simulink model "Nyquistbedingungen"  (Simulink 8.6)
settings: Solver=FixedStepDiscrete  StartTime=0  StopTime=inf  RelTol=1e-3
undefined symbols (not defined in the file or in its folder): dfilt, gcbh, magnitude, rcfiltgaincompat
libraries: commfilt2 x12, commrandsrc2 x6, commdigbbndam3 x4, dspobslib x3, dspstat3 x2, commdigbbndpm3 x2, commchan3 x1, dspsigops x1, simulink x1
CloseFcn:
  | rtwprivate ssgencode ModelCloseRequest Nyquist_Bedingungen
settings Model: Creator=schwall  LastModifiedBy=wunsch
settings DataIOCC: SaveOutput=off  SignalLogging=off  SaveTime=off
settings DebuggingCC: FcnCallInpInsideContextMsg=UseLocalSettings

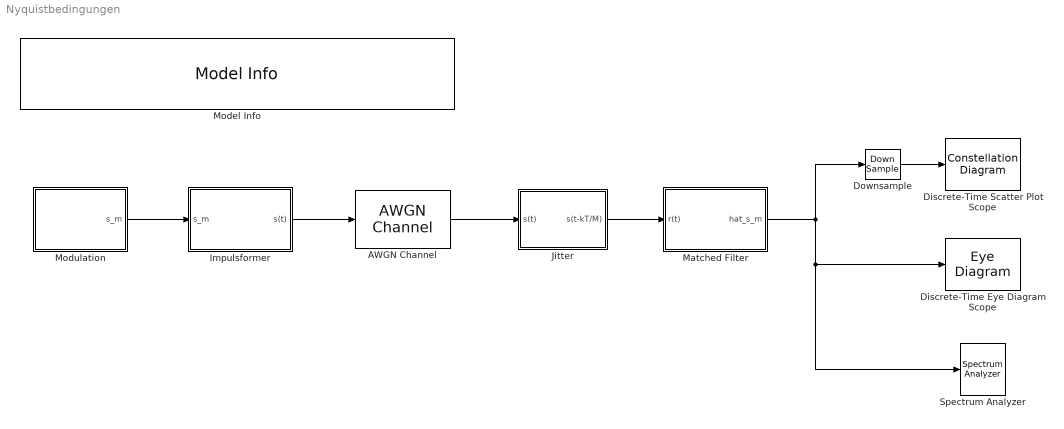
== system Nyquistbedingungen ==
  AWGN Channel : commchan3/AWGN Channel  InputProcessing=Inherited (this choice will be removed - see release notes)  seed=67  noiseMode="Signal to noise ratio  (Es/No)"  EbNodB=10  EsNodB=30  SNRdB=100  bitsPerSym=1  Ps=1/8  Tsym=1/100  variance=1
  Discrete-Time Eye Diagram Scope : EyeDiagram  Tag=EyeDiagram
  Discrete-Time Scatter Plot Scope : ConstellationDiagram  Tag=ScatterPlot
  Downsample : DownSample  N=8
  Impulsformer : Subsystem  mask(Impulsformer){rolloff_set=RRC Rolloff-Faktor 0}
      mask prompts: rolloff_set "Impulsformer:"
      mask help: Impulsformer auswaehlen.
      mask TypeOptions rolloff_set: RRC Rolloff-Faktor 0 | RRC Rolloff-Faktor 0.2 | RRC Rolloff-Faktor 0.4 | RRC Rolloff-Faktor 0.6 | RRC Rolloff-Faktor 0.8 | RRC Rolloff-Faktor 1 | Rechteck-Filter
  Jitter : Subsystem  mask{abtast_set=0}
      mask prompts: abtast_set "Abtastfehler (0...7)"
  Matched Filter : Subsystem  mask(Impulsformer){rolloff_set=RRC Rolloff-Faktor 0}
      mask prompts: rolloff_set "Impulsformer:"
      mask help: Impulsformer auswaehlen.
      mask TypeOptions rolloff_set: RRC Rolloff-Faktor 0 | RRC Rolloff-Faktor 0.2 | RRC Rolloff-Faktor 0.4 | RRC Rolloff-Faktor 0.6 | RRC Rolloff-Faktor 0.8 | RRC Rolloff-Faktor 1 | Rechteck-Filter
  Model Info : simulink/Model-Wide Utilities/Model Info  BlockCM=None  Frame=on  DisplayStringWithTags=|  HorizontalTextAlignment=Left  LeftAlignmentValue=0.02  SourceBlockDiagram=Nyquistbedingungen  TagMaxNumber=20
      | Demo Nyquist Bedingungen
      | Vorlesung Nachrichtentechnik II
      | Institut fuer Nachrichtentechnik (CEL)
  Modulation : Subsystem  mask(Modulation){mod_set=4-QAM, fs=1/100}
      mask prompts: mod_set "Modulationsverfahren:"; fs "Symboldauer [s]"
      mask help: Modulationsverfahren auswaehlen.
      mask TypeOptions mod_set: 2-ASK | QPSK | 16-PSK | 4-QAM | 16-QAM | 256-QAM
  Spectrum Analyzer : SpectrumAnalyzer
  wires:
  Modulation/1(s_m) -> Impulsformer/1(s_m)
  Impulsformer/1(s(t)) -> AWGN Channel/1
  AWGN Channel/1 -> Jitter/1(s(t))
  Downsample/1 -> Discrete-Time Scatter Plot Scope/1
  Matched Filter/1(hat_s_m) -> Downsample/1, Spectrum Analyzer/1, Discrete-Time Eye Diagram Scope/1
  Jitter/1(s(t-kT/M)) -> Matched Filter/1(r(t))

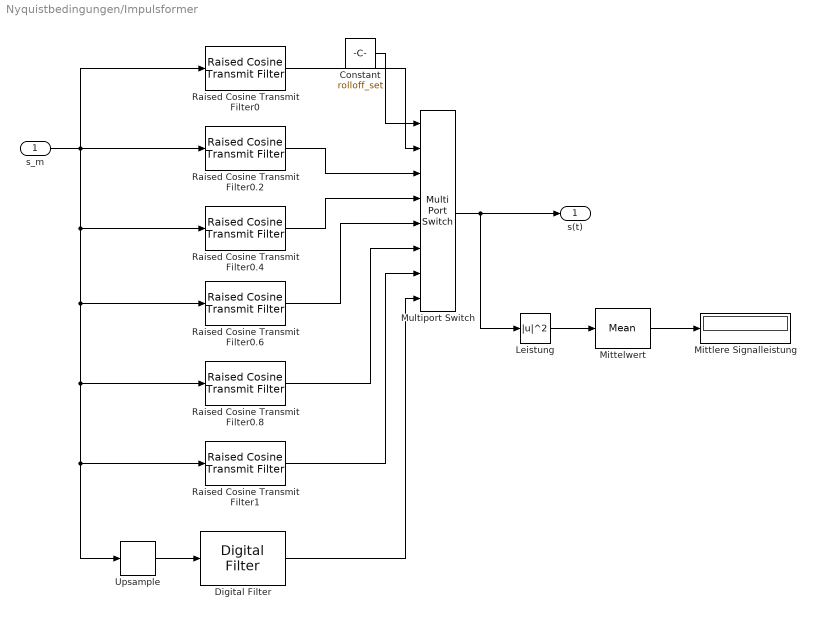
== system Nyquistbedingungen/Impulsformer ==
  s_m : Inport
  Constant : Constant  Value=rolloff_set
  Digital Filter : dspobslib/Digital Filter  TypePopup=FIR (all zeros)  IIRFiltStruct=Direct form II transposed  AllPoleFiltStruct=Direct form  FIRFiltStruct=Direct form  CoeffSource=Specify via dialog  NumCoeffs=1/sqrt(8)*ones(8,1)  DenCoeffs=[1 0.1]  BiQuadCoeffs=[1 0.3 0.4 1 0.1 0.2]  LatticeCoeffs=[0.2 0.4]  denIgnore=on  FiltPerSampPopup=One filter per frame  IC=0  ICnum=0  ICden=0  roundingMode=Floor  overflowMode=off  ScaleValues=1  scaleValueFracLength=14  stageInFracLength=15  stageOutFracLength=15  FilterSource=Specify via dialog  dfiltObjectName=dfilt.dffir([1 2 1])  InputProcessing=Inherited (this choice will be removed - see release notes)
  Leistung : Math  Operator=magnitude^2  SaturateOnIntegerOverflow=on
  Mittelwert : dspstat3/Mean  run=on  reset_popup=None  InputProcessing=Inherited (this choice will be removed - see release notes)  directionMode=Each column  dimension=1  roiEnable=off  roiType=Rectangles  roiPortion=Entire ROI  roiOutput=Individual statistics for each ROI  roiFlag=off  outputDataTypeStr=Inherit: Same as accumulator  outputLastDataTypeStr=Inherit: Same as accumulator  outputMin=[]  outputMax=[]  roundingMode=Floor  overflowMode=off
  Mittlere Signalleistung : Display
  Multiport Switch : MultiPortSwitch  Inputs=7
  Raised Cosine Transmit Filter0 : commfilt2/Raised Cosine Transmit Filter  filtType=Square root  filtSpan=2*(4)  currentFiltSpan=2*(4)  D=4  R=0  sampMode=Mute  saveAsFlag=0  N=8  framing=Maintain input frame rate  InputProcessing=Columns as channels (frame based)  checkGain=User-specified  filterGain=(1)*rcfiltgaincompat(gcbh)  checkCoeff=off  variableName=rcTxFilt  launchFVT=off  roundingMode=Floor  overflowMode=off
  Raised Cosine Transmit Filter0.2 : commfilt2/Raised Cosine Transmit Filter  filtType=Square root  filtSpan=2*(4)  currentFiltSpan=2*(4)  D=4  R=0.2  sampMode=Mute  saveAsFlag=0  N=8  framing=Maintain input frame rate  InputProcessing=Columns as channels (frame based)  checkGain=User-specified  filterGain=(1)*rcfiltgaincompat(gcbh)  checkCoeff=off  variableName=rcTxFilt1  launchFVT=off  roundingMode=Floor  overflowMode=off
  Raised Cosine Transmit Filter0.4 : commfilt2/Raised Cosine Transmit Filter  filtType=Square root  filtSpan=2*(4)  currentFiltSpan=2*(4)  D=4  R=0.4  sampMode=Mute  saveAsFlag=0  N=8  framing=Maintain input frame rate  InputProcessing=Columns as channels (frame based)  checkGain=User-specified  filterGain=(1)*rcfiltgaincompat(gcbh)  checkCoeff=off  variableName=rcTxFilt2  launchFVT=off  roundingMode=Floor  overflowMode=off
  Raised Cosine Transmit Filter0.6 : commfilt2/Raised Cosine Transmit Filter  filtType=Square root  filtSpan=2*(4)  currentFiltSpan=2*(4)  D=4  R=0.6  sampMode=Mute  saveAsFlag=0  N=8  framing=Maintain input frame rate  InputProcessing=Columns as channels (frame based)  checkGain=User-specified  filterGain=(1)*rcfiltgaincompat(gcbh)  checkCoeff=off  variableName=rcTxFilt3  launchFVT=off  roundingMode=Floor  overflowMode=off
  Raised Cosine Transmit Filter0.8 : commfilt2/Raised Cosine Transmit Filter  filtType=Square root  filtSpan=2*(4)  currentFiltSpan=2*(4)  D=4  R=0.8  sampMode=Mute  saveAsFlag=0  N=8  framing=Maintain input frame rate  InputProcessing=Columns as channels (frame based)  checkGain=User-specified  filterGain=(1)*rcfiltgaincompat(gcbh)  checkCoeff=off  variableName=rcTxFilt4  launchFVT=off  roundingMode=Floor  overflowMode=off
  Raised Cosine Transmit Filter1 : commfilt2/Raised Cosine Transmit Filter  filtType=Square root  filtSpan=2*(4)  currentFiltSpan=2*(4)  D=4  R=1  sampMode=Mute  saveAsFlag=0  N=8  framing=Maintain input frame rate  InputProcessing=Columns as channels (frame based)  checkGain=User-specified  filterGain=(1)*rcfiltgaincompat(gcbh)  checkCoeff=off  variableName=rcTxFilt5  launchFVT=off  roundingMode=Floor  overflowMode=off
  Upsample : dspsigops/Upsample  N=8  phase=0  InputProcessing=Inherited (this choice will be removed - see release notes)  RateOptions=Enforce single-rate processing  ic=0  mode=Unused parameter value
  s(t) : Outport
  wires:
  s_m/1 -> Raised Cosine Transmit Filter0/1, Raised Cosine Transmit Filter0.2/1, Raised Cosine Transmit Filter0.4/1, Raised Cosine Transmit Filter0.8/1, Raised Cosine Transmit Filter1/1, Upsample/1, Raised Cosine Transmit Filter0.6/1
  Mittelwert/1 -> Mittlere Signalleistung/1
  Leistung/1 -> Mittelwert/1
  Multiport Switch/1 -> Leistung/1, s(t)/1
  Raised Cosine Transmit Filter0/1 -> Multiport Switch/2
  Raised Cosine Transmit Filter0.2/1 -> Multiport Switch/3
  Raised Cosine Transmit Filter0.4/1 -> Multiport Switch/4
  Raised Cosine Transmit Filter0.6/1 -> Multiport Switch/5
  Raised Cosine Transmit Filter0.8/1 -> Multiport Switch/6
  Raised Cosine Transmit Filter1/1 -> Multiport Switch/7
  Constant/1 -> Multiport Switch/1
  Digital Filter/1 -> Multiport Switch/8
  Upsample/1 -> Digital Filter/1

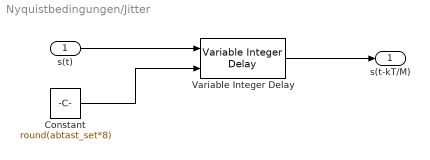
== system Nyquistbedingungen/Jitter ==
  s(t) : Inport
  Constant : Constant  Value=round(abtast_set*8)
  Variable Integer Delay : dspobslib/Variable Integer Delay  dmax=7  InputProcessing=Inherited (this choice will be removed - see release notes)  ic=0  noDFT=off
  s(t-kT/M) : Outport
  wires:
  Variable Integer Delay/1 -> s(t-kT/M)/1
  Constant/1 -> Variable Integer Delay/2
  s(t)/1 -> Variable Integer Delay/1

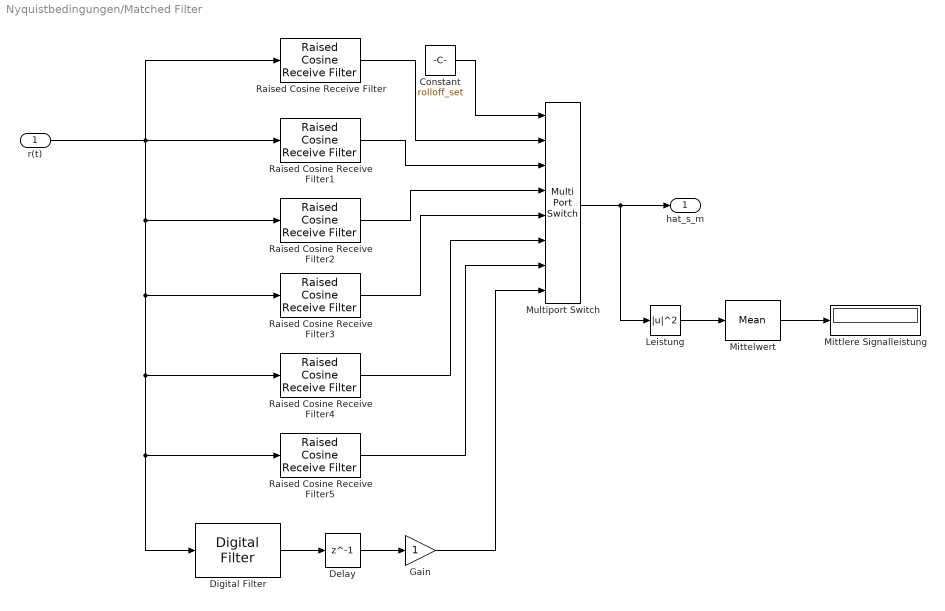
== system Nyquistbedingungen/Matched Filter ==
  r(t) : Inport
  Constant : Constant  Value=rolloff_set
  Delay : Delay  DelayLength=1  InitialCondition=0  InputProcessing=Columns as channels (frame based)
  Digital Filter : dspobslib/Digital Filter  TypePopup=FIR (all zeros)  IIRFiltStruct=Direct form II transposed  AllPoleFiltStruct=Direct form  FIRFiltStruct=Direct form  CoeffSource=Specify via dialog  NumCoeffs=1/sqrt(8)*ones(8,1)  DenCoeffs=[1 0.1]  BiQuadCoeffs=[1 0.3 0.4 1 0.1 0.2]  LatticeCoeffs=[0.2 0.4]  denIgnore=on  FiltPerSampPopup=One filter per frame  IC=0  ICnum=0  ICden=0  roundingMode=Floor  overflowMode=off  ScaleValues=1  scaleValueFracLength=14  stageInFracLength=15  stageOutFracLength=15  FilterSource=Specify via dialog  dfiltObjectName=dfilt.dffir([1 2 1])  InputProcessing=Inherited (this choice will be removed - see release notes)
  Gain : Gain
  Leistung : Math  Operator=magnitude^2  SaturateOnIntegerOverflow=on
  Mittelwert : dspstat3/Mean  run=on  reset_popup=None  InputProcessing=Inherited (this choice will be removed - see release notes)  directionMode=Each column  dimension=1  roiEnable=off  roiType=Rectangles  roiPortion=Entire ROI  roiOutput=Individual statistics for each ROI  roiFlag=off  outputDataTypeStr=Inherit: Same as accumulator  outputLastDataTypeStr=Inherit: Same as accumulator  outputMin=[]  outputMax=[]  roundingMode=Floor  overflowMode=off
  Mittlere Signalleistung : Display
  Multiport Switch : MultiPortSwitch  Inputs=7
  Raised Cosine Receive Filter : commfilt2/Raised Cosine Receive Filter  filtType=Square root  N=8  filtSpan=2*(4)  currentFiltSpan=2*(4)  D=4  R=0  sampMode=Mute  saveAsFlag=0  rateMode=Downsampling  downFactor=1  downOffset=0  framing=Maintain input frame rate  InputProcessing=Columns as channels (frame based)  checkGain=User-specified  filterGain=(1)*rcfiltgaincompat(gcbh)  checkCoeff=off  variableName=rcRxFilt  launchFVT=off  roundingMode=Floor  overflowMode=off
  Raised Cosine Receive Filter1 : commfilt2/Raised Cosine Receive Filter  filtType=Square root  N=8  filtSpan=2*(4)  currentFiltSpan=2*(4)  D=4  R=0.2  sampMode=Mute  saveAsFlag=0  rateMode=Downsampling  downFactor=1  downOffset=0  framing=Maintain input frame rate  InputProcessing=Columns as channels (frame based)  checkGain=User-specified  filterGain=(1)*rcfiltgaincompat(gcbh)  checkCoeff=off  variableName=rcRxFilt1  launchFVT=off  roundingMode=Floor  overflowMode=off
  Raised Cosine Receive Filter2 : commfilt2/Raised Cosine Receive Filter  filtType=Square root  N=8  filtSpan=2*(4)  currentFiltSpan=2*(4)  D=4  R=0.4  sampMode=Mute  saveAsFlag=0  rateMode=Downsampling  downFactor=1  downOffset=0  framing=Maintain input frame rate  InputProcessing=Columns as channels (frame based)  checkGain=User-specified  filterGain=(1)*rcfiltgaincompat(gcbh)  checkCoeff=off  variableName=rcRxFilt2  launchFVT=off  roundingMode=Floor  overflowMode=off
  Raised Cosine Receive Filter3 : commfilt2/Raised Cosine Receive Filter  filtType=Square root  N=8  filtSpan=2*(4)  currentFiltSpan=2*(4)  D=4  R=0.6  sampMode=Mute  saveAsFlag=0  rateMode=Downsampling  downFactor=1  downOffset=0  framing=Maintain input frame rate  InputProcessing=Columns as channels (frame based)  checkGain=User-specified  filterGain=(1)*rcfiltgaincompat(gcbh)  checkCoeff=off  variableName=rcRxFilt3  launchFVT=off  roundingMode=Floor  overflowMode=off
  Raised Cosine Receive Filter4 : commfilt2/Raised Cosine Receive Filter  filtType=Square root  N=8  filtSpan=2*(4)  currentFiltSpan=2*(4)  D=4  R=0.8  sampMode=Mute  saveAsFlag=0  rateMode=Downsampling  downFactor=1  downOffset=0  framing=Maintain input frame rate  InputProcessing=Columns as channels (frame based)  checkGain=User-specified  filterGain=(1)*rcfiltgaincompat(gcbh)  checkCoeff=off  variableName=rcRxFilt4  launchFVT=off  roundingMode=Floor  overflowMode=off
  Raised Cosine Receive Filter5 : commfilt2/Raised Cosine Receive Filter  filtType=Square root  N=8  filtSpan=2*(4)  currentFiltSpan=2*(4)  D=4  R=1  sampMode=Mute  saveAsFlag=0  rateMode=Downsampling  downFactor=1  downOffset=0  framing=Maintain input frame rate  InputProcessing=Columns as channels (frame based)  checkGain=User-specified  filterGain=(1)*rcfiltgaincompat(gcbh)  checkCoeff=off  variableName=rcRxFilt5  launchFVT=off  roundingMode=Floor  overflowMode=off
  hat_s_m : Outport
  wires:
  Raised Cosine Receive Filter5/1 -> Multiport Switch/7
  Raised Cosine Receive Filter4/1 -> Multiport Switch/6
  Raised Cosine Receive Filter3/1 -> Multiport Switch/5
  Raised Cosine Receive Filter2/1 -> Multiport Switch/4
  Constant/1 -> Multiport Switch/1
  Multiport Switch/1 -> Leistung/1, hat_s_m/1
  Leistung/1 -> Mittelwert/1
  Mittelwert/1 -> Mittlere Signalleistung/1
  r(t)/1 -> Raised Cosine Receive Filter4/1, Raised Cosine Receive Filter5/1, Digital Filter/1, Raised Cosine Receive Filter3/1, Raised Cosine Receive Filter2/1, Raised Cosine Receive Filter/1, Raised Cosine Receive Filter1/1
  Raised Cosine Receive Filter/1 -> Multiport Switch/2
  Raised Cosine Receive Filter1/1 -> Multiport Switch/3
  Digital Filter/1 -> Delay/1
  Gain/1 -> Multiport Switch/8
  Delay/1 -> Gain/1

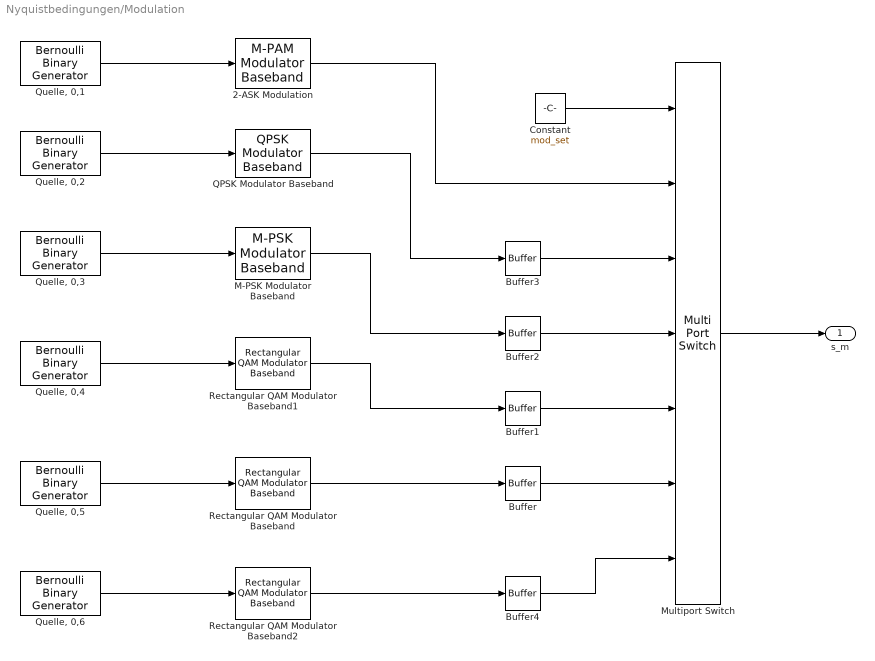
== system Nyquistbedingungen/Modulation ==
  2-ASK Modulation : commdigbbndam3/M-PAM Modulator Baseband  M=2  InType=Integer  Enc=Binary  PowType=Average Power  MinDist=2  AvgPow=1  PeakPow=1  outDtype=double  outWordLen=16  outUDDataType=sfix(16)  outFracLenMode=Best precision  outFracLen=15
  Buffer{,1..4} (5 alike) : Buffer  N=8
  Constant : Constant  Value=mod_set
  M-PSK Modulator Baseband : commdigbbndpm3/M-PSK Modulator Baseband  M=16  InType=Bit  Enc=Gray  Mapping=[0:7]  Ph=pi/8  outDtype=double  outWordLen=16  outUDDataType=sfix(16)  outFracLenMode=Best precision  outFracLen=15
  Multiport Switch : MultiPortSwitch  Inputs=6
  QPSK Modulator Baseband : commdigbbndpm3/QPSK Modulator Baseband  InType=Bit  Enc=Gray  Ph=0  outDtype=double  outWordLen=16  outUDDataType=sfix(16)  outFracLenMode=Best precision  outFracLen=15
  "Quelle, 0,1" : commrandsrc2/Bernoulli Binary Generator  P=0.5  seed=61  Ts=8*fs/8  frameBased=on  sampPerFrame=8  orient=off  outDataType=double
  "Quelle, 0,2" : commrandsrc2/Bernoulli Binary Generator  P=0.5  seed=61  Ts=4*fs/8  frameBased=on  sampPerFrame=8  orient=off  outDataType=double
  "Quelle, 0,3" : commrandsrc2/Bernoulli Binary Generator  P=0.5  seed=61  Ts=2*fs/8  frameBased=on  sampPerFrame=8  orient=off  outDataType=double
  "Quelle, 0,4" : commrandsrc2/Bernoulli Binary Generator  P=0.5  seed=61  Ts=4*fs/8  frameBased=on  sampPerFrame=8  orient=off  outDataType=double
  "Quelle, 0,5" : commrandsrc2/Bernoulli Binary Generator  P=0.5  seed=61  Ts=2*fs/8  frameBased=on  sampPerFrame=8  orient=off  outDataType=double
  "Quelle, 0,6" : commrandsrc2/Bernoulli Binary Generator  P=0.5  seed=61  Ts=fs/8  frameBased=on  sampPerFrame=8  orient=off  outDataType=double
  Rectangular QAM Modulator Baseband : commdigbbndam3/Rectangular QAM Modulator Baseband  M=16  InType=Bit  Enc=Gray  Mapping=[0:15]  PowType=Average Power  MinDist=2  AvgPow=1  PeakPow=1  Ph=0  outDtype=double  outWordLen=16  outUDDataType=sfix(16)  outFracLenMode=Best precision  outFracLen=15
  Rectangular QAM Modulator Baseband1 : commdigbbndam3/Rectangular QAM Modulator Baseband  M=4  InType=Bit  Enc=Gray  Mapping=[0:15]  PowType=Average Power  MinDist=2  AvgPow=1  PeakPow=1  Ph=0  outDtype=double  outWordLen=16  outUDDataType=sfix(16)  outFracLenMode=Best precision  outFracLen=15
  Rectangular QAM Modulator Baseband2 : commdigbbndam3/Rectangular QAM Modulator Baseband  M=256  InType=Bit  Enc=Gray  Mapping=[0:15]  PowType=Average Power  MinDist=2  AvgPow=1  PeakPow=1  Ph=0  outDtype=double  outWordLen=16  outUDDataType=sfix(16)  outFracLenMode=Best precision  outFracLen=15
  s_m : Outport
  wires:
  2-ASK Modulation/1 -> Multiport Switch/2
  QPSK Modulator Baseband/1 -> Buffer3/1
  M-PSK Modulator Baseband/1 -> Buffer2/1
  Rectangular QAM Modulator Baseband1/1 -> Buffer1/1
  Rectangular QAM Modulator Baseband/1 -> Buffer/1
  Constant/1 -> Multiport Switch/1
  Multiport Switch/1 -> s_m/1
  "Quelle, 0,1"/1 -> 2-ASK Modulation/1
  "Quelle, 0,2"/1 -> QPSK Modulator Baseband/1
  "Quelle, 0,3"/1 -> M-PSK Modulator Baseband/1
  "Quelle, 0,4"/1 -> Rectangular QAM Modulator Baseband1/1
  "Quelle, 0,5"/1 -> Rectangular QAM Modulator Baseband/1
  Buffer/1 -> Multiport Switch/6
  Buffer1/1 -> Multiport Switch/5
  Buffer2/1 -> Multiport Switch/4
  Buffer3/1 -> Multiport Switch/3
  Rectangular QAM Modulator Baseband2/1 -> Buffer4/1
  "Quelle, 0,6"/1 -> Rectangular QAM Modulator Baseband2/1
  Buffer4/1 -> Multiport Switch/7
